simulink model "Seesaw_Validation"  (R2025b)
settings: Solver=FixedStepDiscrete  StartTime=0.0  StopTime=290  FixedStep=0.002  RelTol=1e-3
undefined symbols (not defined in the file): alpha_f, HIL, K_E_SW, K_ec, K_gs, K_hw, V_sat
libraries: quarc_library x4
settings Model: Creator=U448565  LastModifiedBy=U448565

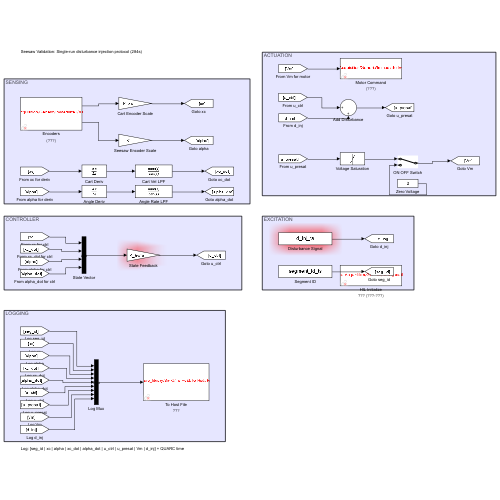
[thumbnail: Simulink's stored preview of the top-level diagram]
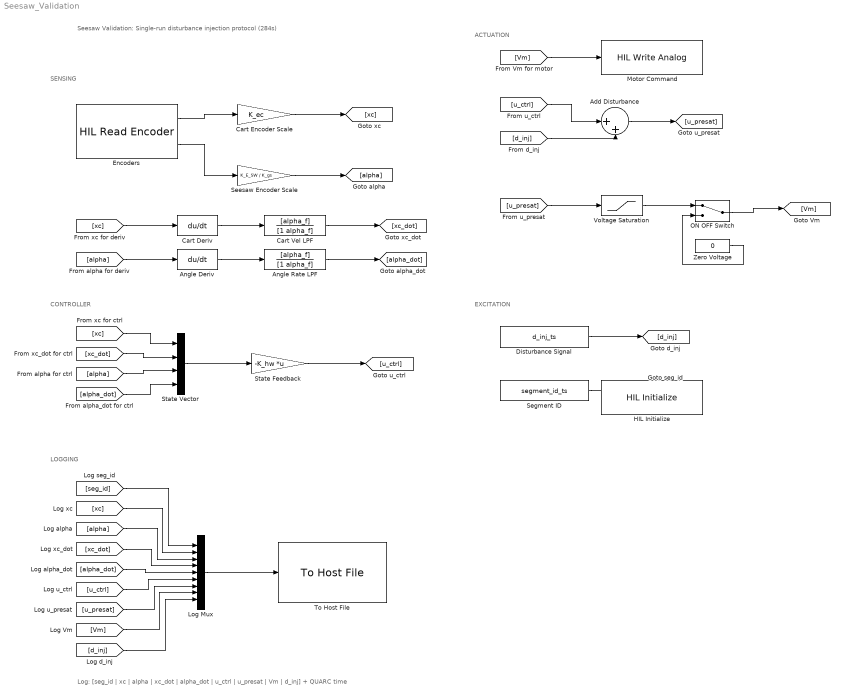
== system Seesaw_Validation ==
  note: SENSING
  note: CONTROLLER
  note: EXCITATION
  note: ACTUATION
  note: LOGGING
  note: Log: [seg_id | xc | alpha | xc_dot | alpha_dot | u_ctrl | u_presat | Vm | d_inj] + QUARC time
  note: Seesaw Validation: Single-run disturbance injection protocol (284s)
  Add Disturbance : Sum  Inputs=|++
  Angle Deriv : Derivative
  Angle Rate LPF : TransferFcn  Numerator=[alpha_f]  Denominator=[1 alpha_f]
  Cart Deriv : Derivative
  Cart Encoder Scale : Gain  Gain=K_ec
  Cart Vel LPF : TransferFcn  Numerator=[alpha_f]  Denominator=[1 alpha_f]
  Disturbance Signal : FromWorkspace  VariableName=d_inj_ts
  Encoders : quarc_library/Data Acquisition/Generic/Immediate I//O/HIL Read Encoder  object_name=HIL-1  channels=[0:1]  sample_time=qc_get_step_size  active=on  vector_output=off  data_type_mode=Inherit via back propagation  data_type=double
  HIL Initialize : quarc_library/Data Acquisition/Generic/Configuration/HIL Initialize  object_name=HIL-1  board_type=q2_usb  board_number=0  board_options=d0=digital;d1=digital;led=auto;update_rate=normal  exclusive=off  active=off  hardware_clocks=[0:2]  clock_modes=[]  initial_clock_frequencies=[]  set_clock_params_at_start=off  set_clock_params_at_switch_in=off  set_clock_frequencies_at_start=off  set_clock_frequencies_at_switch_in=off  analog_input_channels=[0:1]  analog_input_configurations=[]  analog_input_maximums=10  analog_input_minimums=-10  set_analog_input_params_at_start=on  set_analog_input_params_at_switch_in=off  analog_output_channels=[0:1]  analog_output_maximums=10  analog_output_minimums=-10  initial_analog_outputs=[0]  final_analog_outputs=[0]  watchdog_analog_outputs=0  set_analog_output_params_at_start=on  set_analog_output_params_at_switch_in=off  set_analog_outputs_at_start=on  set_analog_outputs_at_switch_in=off  set_analog_outputs_at_terminate=on  set_analog_outputs_at_switch_out=off  set_analog_outputs_on_watchdog=off  digital_input_channels=[]  digital_output_channels=[0:7]  digital_output_configuration=[]  initial_digital_outputs=[0]  final_digital_outputs=[0]  watchdog_digital_outputs=[0]  set_digital_output_params_at_start=off  set_digital_output_params_at_switch_in=off  set_digital_outputs_at_start=on  set_digital_outputs_at_switch_in=off  set_digital_outputs_at_terminate=on  set_digital_outputs_at_switch_out=off  set_digital_outputs_on_watchdog=off  encoder_channels=[0:1]  quadrature=[4]  encoder_filter_frequency=[]  initial_encoder_counts=[0]  set_encoder_params_at_start=on  set_encoder_params_at_switch_in=off  set_encoder_counts_at_start=on  set_encoder_counts_at_switch_in=off  pwm_channels=[]  pwm_modes=[0]  pwm_frequency=1/0.020  pwm_configuration=[]  pwm_alignment=[]  pwm_polarity=[]  pwm_leading_deadband=[]  pwm_trailing_deadband=[]  initial_pwm_outputs=[0]  final_pwm_outputs=[0]  watchdog_pwm_outputs=[0]  set_pwm_params_at_start=on  set_pwm_params_at_switch_in=off  set_pwm_outputs_at_start=on  set_pwm_outputs_at_switch_in=off  set_pwm_outputs_at_terminate=on  set_pwm_outputs_at_switch_out=off  set_pwm_outputs_on_watchdog=off  other_output_channels=[]  initial_other_outputs=[]  final_other_outputs=[]  watchdog_other_outputs=[]  set_other_outputs_at_start=off  set_other_outputs_at_switch_in=off  set_other_outputs_at_terminate=off  set_other_outputs_at_switch_out=off  set_other_outputs_on_watchdog=off
  Log Mux : Mux  Inputs=9
  Motor Command : quarc_library/Data Acquisition/Generic/Immediate I//O/HIL Write Analog  object_name=HIL-1  channels=0  sample_time=-1  active=off  vector_input=off
  ON OFF Switch : ManualSwitch
  Seesaw Encoder Scale : Gain  Gain=K_E_SW / K_gs
  Segment ID : FromWorkspace  VariableName=segment_id_ts
  State Feedback : Gain  Gain=-K_hw  Multiplication=Matrix(K*u)
  State Vector : Mux
  To Host File : quarc_library/Sinks/To Host/To Host File  source=Specify via dialog (do not evaluate)  file_name=data_%{date}_%{time}.mat  variable_name=data  decimation=1  sample_time=-1  file_format=MAT-file v.4  options=No header or footer  append=off  final_file_name=data_05-May-2026_17-28-00.mat  encoding=Default  bitrate=0
  Voltage Saturation : Saturate  UpperLimit=V_sat  LowerLimit=-V_sat
  Zero Voltage : Constant  Value=0
  wires:
  Encoders/1 -> Cart Encoder Scale/1
  Encoders/2 -> Seesaw Encoder Scale/1
  Cart Encoder Scale/1 -> [xc]
  Seesaw Encoder Scale/1 -> [alpha]
  [xc] -> Cart Deriv/1
  [alpha] -> Angle Deriv/1
  Cart Deriv/1 -> Cart Vel LPF/1
  Angle Deriv/1 -> Angle Rate LPF/1
  Cart Vel LPF/1 -> [xc_dot]
  Angle Rate LPF/1 -> [alpha_dot]
  [xc] -> State Vector/1
  [xc_dot] -> State Vector/2
  [alpha] -> State Vector/3
  [alpha_dot] -> State Vector/4
  State Vector/1 -> State Feedback/1
  State Feedback/1 -> [u_ctrl]
  Disturbance Signal/1 -> [d_inj]
  Segment ID/1 -> [seg_id]
  [u_ctrl] -> Add Disturbance/1
  [d_inj] -> Add Disturbance/2
  Add Disturbance/1 -> [u_presat]
  [u_presat] -> Voltage Saturation/1
  Voltage Saturation/1 -> ON OFF Switch/1
  Zero Voltage/1 -> ON OFF Switch/2
  ON OFF Switch/1 -> [Vm]
  [Vm] -> Motor Command/1
  [seg_id] -> Log Mux/1
  [xc] -> Log Mux/2
  [alpha] -> Log Mux/3
  [xc_dot] -> Log Mux/4
  [alpha_dot] -> Log Mux/5
  [u_ctrl] -> Log Mux/6
  [u_presat] -> Log Mux/7
  [Vm] -> Log Mux/8
  [d_inj] -> Log Mux/9
  Log Mux/1 -> To Host File/1
